simulink model "simulink_model_mbpo"  (R2022b)
settings: Solver=VariableStepAuto  StartTime=0.0  StopTime=5  FixedStep=1.0  RelTol=1e-3
values from neighbouring files (symbols this model uses):
  aa = (((m*l)^2)*g)/AA    (= 0.275046740282)    [createagent_mbpo.m]
  bb = (I +m*(l^2))*c/AA    (= 0.588785047389)    [createagent_mbpo.m]
  cc = (b*m*l)/AA    (= 4.42542074273e-05)    [createagent_mbpo.m]
  dd = (m*g*l*(M+m))/AA    (= 6.05102828621)    [createagent_mbpo.m]
  ee = (m*l*c)/AA    (= 0.353271042564)    [createagent_mbpo.m]
  ff = ((M+m)*b)/AA    (= 0.0009735925634)    [createagent_mbpo.m]
  mm = (I +m*(l^2))/AA    (= 0.9345794403)    [createagent_mbpo.m]
  nn = (m*l)/AA    (= 0.56074768661)    [createagent_mbpo.m]
  oo = (2*l)/AA    (= 11.2149537322)    [createagent_mbpo.m]
  thetastartdelta = 0    [createagent_mbpo.m]
  xstartdelta = 0    [createagent_mbpo.m]
libraries: rllib x1
settings Model: Creator=Wolfgang  LastModifiedBy=Wolfgang

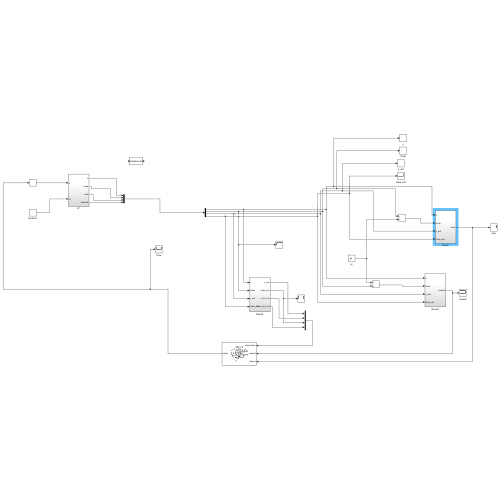
[thumbnail: Simulink's stored preview of the top-level diagram]
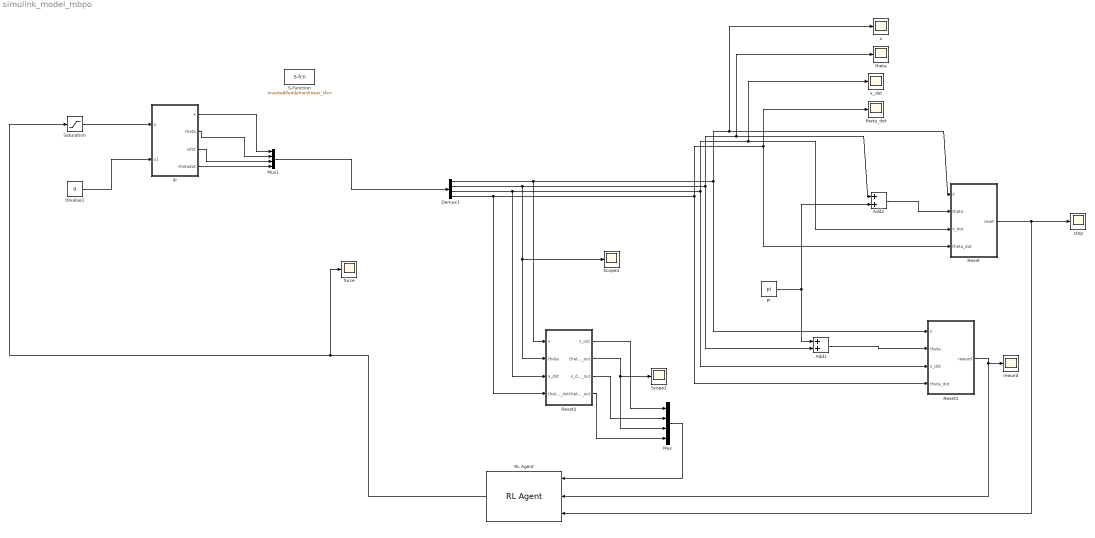
== system simulink_model_mbpo ==
  Add1 : Sum
  Add2 : Sum
  Demux1 : Demux
  IP : Subsystem
  Mux : Mux
  Mux1 : Mux
  RL Agent : rllib/RL Agent  Agent=agent  ExternalActionAsInput=off  ProvideLastAction=off  ProvideCumRwd=off  TreatAsDirectFeedthrough=on  UseStrictObservationDataTypes=off
  Reset : Subsystem
  Reset1 : Subsystem
  Reset2 : Subsystem
  S-Function : S-Function  FunctionName=invertedPendelnonlinear_sfcn  Parameters=xstart; thetastart; 0; 0  SFunctionDeploymentMode=off  EnableBusSupport=off
  Saturation : Saturate  UpperLimit=1000  LowerLimit=-1000
  Scope2 : Scope
  Scope4 : Scope
  force : Scope
  pi : Constant  Tag=tt  Value=pi
  reward : Scope
  stop : Scope
  t0value1 : Constant  Tag=tt  Value=0
  theta : Scope
  theta_dot : Scope
  x : Scope
  x_dot : Scope
  wires:
  Demux1/2 -> Scope4/1, Reset2/2(theta), Add1/2, Add2/1, theta/1
  Demux1/3 -> Reset2/3(x_dot), x_dot/1, Reset/3(x_dot), Reset1/3(x_dot)
  Demux1/4 -> Reset2/4(theta_dot), Reset/4(theta_dot), theta_dot/1, Reset1/4(theta_dot)
  Reset/1(reset) -> RL Agent/3, stop/1
  Reset1/1(reward) -> RL Agent/2, reward/1
  RL Agent/1 -> Saturation/1, force/1
  Mux/1 -> RL Agent/1
  Reset2/1(x_out) -> Mux/1
  Reset2/3(x_dot_out) -> Mux/2
  Reset2/2(theta_out) -> Scope2/1, Mux/3
  Reset2/4(theta_dot_out) -> Mux/4
  IP/1(x) -> Mux1/1
  Mux1/1 -> Demux1/1
  IP/3(xdot) -> Mux1/3
  IP/4(thetadot) -> Mux1/4
  t0value1/1 -> IP/2(u1)
  IP/2(theta) -> Mux1/2
  Demux1/1 -> Reset1/1(x), x/1, Reset/1(x), Reset2/1(x)
  Add1/1 -> Reset1/2(theta)
  Add2/1 -> Reset/2(theta)
  pi/1 -> Add2/2, Add1/1
  Saturation/1 -> IP/1(u)

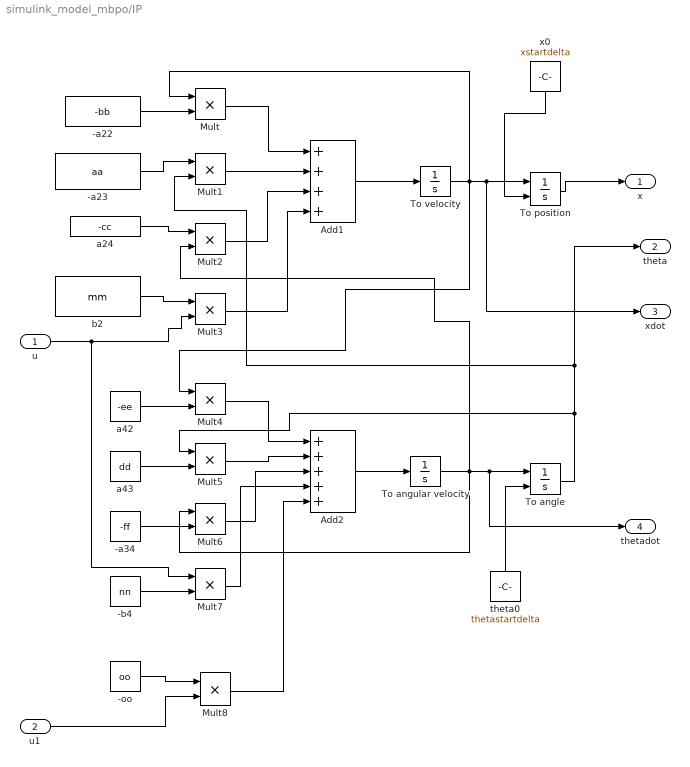
== system simulink_model_mbpo/IP ==
  u : Inport
  u1 : Inport  Port=2
  -a22 : Constant  Value=-bb
  -a23 : Constant  Value=aa
  -a34 : Constant  Value=-ff
  -b4 : Constant  Value=nn
  -oo : Constant  Value=oo
  Add1 : Sum  Inputs=++++
  Add2 : Sum  Inputs=+++++
  Mult{,1..8} (9 alike) : Product  Inputs=**
  To angle : Integrator  InitialConditionSource=external  InitialCondition=1.5
  To angular velocity : Integrator
  To position : Integrator  InitialConditionSource=external  InitialCondition=1
  To velocity : Integrator
  a24 : Constant  Value=-cc
  a42 : Constant  Value=-ee
  a43 : Constant  Value=dd
  b2 : Constant  Value=mm
  theta0 : Constant  Value=thetastartdelta
  x0 : Constant  Value=xstartdelta
  x : Outport  VectorParamsAs1DForOutWhenUnconnected=off
  theta : Outport  Port=2  VectorParamsAs1DForOutWhenUnconnected=off
  xdot : Outport  Port=3  VectorParamsAs1DForOutWhenUnconnected=off
  thetadot : Outport  Port=4  VectorParamsAs1DForOutWhenUnconnected=off
  wires:
  u1/1 -> Mult8/2
  -oo/1 -> Mult8/1
  Mult8/1 -> Add2/5
  x0/1 -> To position/2
  theta0/1 -> To angle/2
  To position/1 -> x/1
  a24/1 -> Mult2/1
  Mult5/1 -> Add2/2
  Mult/1 -> Add1/1
  a42/1 -> Mult4/2
  u/1 -> Mult3/2, Mult7/1
  Mult2/1 -> Add1/3
  Mult4/1 -> Add2/1
  a43/1 -> Mult5/2
  Mult7/1 -> Add2/4
  To angle/1 -> Mult5/1, Mult1/2, theta/1
  To velocity/1 -> To position/1, xdot/1, Mult/1, Mult4/1
  -a23/1 -> Mult1/1
  To angular velocity/1 -> To angle/1, thetadot/1, Mult2/2, Mult6/1
  b2/1 -> Mult3/1
  Add1/1 -> To velocity/1
  Mult1/1 -> Add1/2
  Mult3/1 -> Add1/4
  Mult6/1 -> Add2/3
  -b4/1 -> Mult7/2
  -a34/1 -> Mult6/2
  Add2/1 -> To angular velocity/1
  -a22/1 -> Mult/2

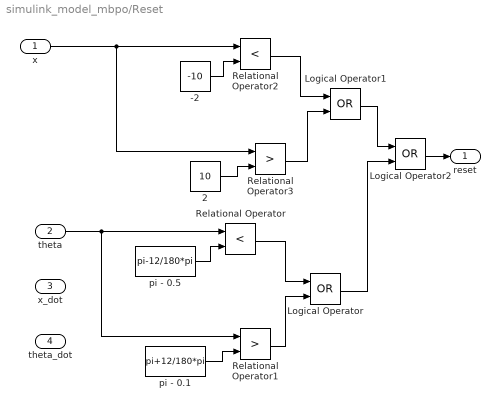
== system simulink_model_mbpo/Reset ==
  x : Inport
  theta : Inport  Port=2
  x_dot : Inport  Port=3
  theta_dot : Inport  Port=4
  -2 : Constant  Value=-10
  2 : Constant  Value=10
  Logical Operator : Logic  Operator=OR  AllPortsSameDT=off  OutDataTypeStr=boolean
  Logical Operator1 : Logic  Operator=OR  AllPortsSameDT=off  OutDataTypeStr=boolean
  Logical Operator2 : Logic  Operator=OR  AllPortsSameDT=off  OutDataTypeStr=boolean
  Relational Operator : RelationalOperator  Operator=<  OutDataTypeStr=boolean  RndMeth=Simplest  InputSameDT=off
  Relational Operator1 : RelationalOperator  Operator=>  OutDataTypeStr=boolean  RndMeth=Simplest  InputSameDT=off
  Relational Operator2 : RelationalOperator  Operator=<  OutDataTypeStr=boolean  RndMeth=Simplest  InputSameDT=off
  Relational Operator3 : RelationalOperator  Operator=>  OutDataTypeStr=boolean  RndMeth=Simplest  InputSameDT=off
  pi - 0.1 : Constant  Value=pi+12/180*pi
  pi - 0.5 : Constant  Value=pi-12/180*pi
  reset : Outport  VectorParamsAs1DForOutWhenUnconnected=off
  wires:
  theta/1 -> Relational Operator1/1, Relational Operator/1
  pi - 0.5/1 -> Relational Operator/2
  Relational Operator/1 -> Logical Operator/1
  pi - 0.1/1 -> Relational Operator1/2
  Logical Operator2/1 -> reset/1
  Relational Operator1/1 -> Logical Operator/2
  Relational Operator3/1 -> Logical Operator1/2
  Relational Operator2/1 -> Logical Operator1/1
  -2/1 -> Relational Operator2/2
  2/1 -> Relational Operator3/2
  x/1 -> Relational Operator3/1, Relational Operator2/1
  Logical Operator1/1 -> Logical Operator2/1
  Logical Operator/1 -> Logical Operator2/2

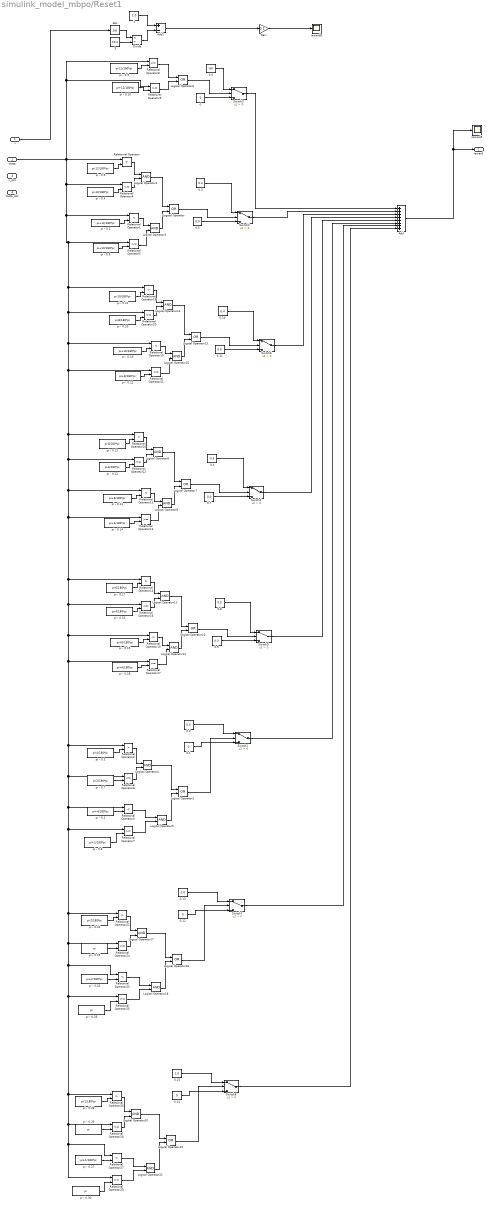
== system simulink_model_mbpo/Reset1 ==
  x : Inport
  theta : Inport  Port=2
  x_dot : Inport  Port=3
  theta_dot : Inport  Port=4
  -1 : Constant  Value=0
  0.1 : Constant  Value=0
  0.10 : Constant  Value=0.4
  0.{5,7,9,11} (4 alike) : Constant  Value=0.0
  0.12 : Constant  Value=0
  0.13 : Constant  Value=0.6
  0.14 : Constant  Value=0
  0.15 : Constant  Value=1.0
  0.2 : Constant  Value=0.5
  0.3 : Constant  Value=0.3
  0.4 : Constant  Value=0.5
  0.6 : Constant  Value=-50
  0.8 : Constant  Value=0.5
  1 : Constant  Value=1.0
  3 : Constant  Value=10.0
  Abs : Abs  SaturateOnIntegerOverflow=off
  Add : Sum  Inputs=++++++++
  Add1 : Sum  Inputs=+-
  Divide : Product  Inputs=*/
  Gain : Gain  Gain=0.1
  Logical Operator{,1,6..7,10,13,16,19} (8 alike) : Logic  Operator=OR  AllPortsSameDT=off  OutDataTypeStr=boolean
  Logical Operator{2..5,8..9,11..12,14..15,17..18,20..21} (14 alike) : Logic  AllPortsSameDT=off  OutDataTypeStr=boolean
  Relational Operator{,2,10,14,18,22,26} (7 alike) : RelationalOperator  Operator=>  OutDataTypeStr=boolean  RndMeth=Simplest  InputSameDT=off
  Relational Operator{1,3,11,15,19,23,27} (7 alike) : RelationalOperator  Operator=<  OutDataTypeStr=boolean  RndMeth=Simplest  InputSameDT=off
  Relational Operator{4,6,8,12,16,20,24,28} (8 alike) : RelationalOperator  Operator=<=  OutDataTypeStr=boolean  RndMeth=Simplest  InputSameDT=off
  Relational Operator{5,7,9,13,17,21,25,29} (8 alike) : RelationalOperator  OutDataTypeStr=boolean  RndMeth=Simplest  InputSameDT=off
  Switch{1..8} (8 alike) : Switch  Criteria=u2 > Threshold  SaturateOnIntegerOverflow=off  InputSameDT=off
  pi - 0.1 : Constant  Value=pi+12/180*pi
  pi - 0.10 : Constant  Value=pi+12/180*pi
  pi - 0.11 : Constant  Value=pi+8/180*pi
  pi - 0.12 : Constant  Value=pi-6/180*pi
  pi - 0.13 : Constant  Value=pi-8/180*pi
  pi - 0.14 : Constant  Value=pi+6/180*pi
  pi - 0.15 : Constant  Value=pi+6/180*pi
  pi - 0.16 : Constant  Value=pi-4/180*pi
  pi - 0.17 : Constant  Value=pi-6/180*pi
  pi - 0.18 : Constant  Value=pi+4/180*pi
  pi - 0.19 : Constant  Value=pi+10/180*pi
  pi - 0.2 : Constant  Value=pi+4/180*pi
  pi - 0.20 : Constant  Value=pi-8/180*pi
  pi - 0.21 : Constant  Value=pi-10/180*pi
  pi - 0.22 : Constant  Value=pi+8/180*pi
  pi - 0.23 : Constant  Value=pi+2/180*pi
  pi - 0.24 : Constant  Value=pi-2/180*pi
  pi - 0.{25..26,29..30} (4 alike) : Constant  Value=pi
  pi - 0.27 : Constant  Value=pi+1/180*pi
  pi - 0.28 : Constant  Value=pi-1/180*pi
  pi - 0.3 : Constant  Value=pi-4/180*pi
  pi - 0.4 : Constant  Value=pi-10/180*pi
  pi - 0.5 : Constant  Value=pi-12/180*pi
  pi - 0.6 : Constant  Value=pi+10/180*pi
  pi - 0.7 : Constant  Value=pi-2/180*pi
  pi - 0.8 : Constant  Value=pi+2/180*pi
  pi - 0.9 : Constant  Value=pi-12/180*pi
  reward5 : Scope
  reward8 : Scope
  reward : Outport  VectorParamsAs1DForOutWhenUnconnected=off
  wires:
  pi - 0.5/1 -> Relational Operator/2
  Relational Operator/1 -> Logical Operator2/1
  pi - 0.1/1 -> Relational Operator1/2
  pi - 0.2/1 -> Relational Operator3/2
  Relational Operator3/1 -> Logical Operator5/1
  pi - 0.3/1 -> Relational Operator2/2
  Logical Operator1/1 -> Switch1/2
  pi - 0.4/1 -> Relational Operator4/2
  Relational Operator4/1 -> Logical Operator2/2
  pi - 0.6/1 -> Relational Operator5/2
  Relational Operator5/1 -> Logical Operator3/2
  Relational Operator1/1 -> Logical Operator3/1
  Logical Operator3/1 -> Logical Operator/2
  Logical Operator2/1 -> Logical Operator/1
  pi - 0.7/1 -> Relational Operator6/2
  Relational Operator6/1 -> Logical Operator4/2
  Relational Operator2/1 -> Logical Operator4/1
  pi - 0.8/1 -> Relational Operator7/2
  Relational Operator7/1 -> Logical Operator5/2
  Logical Operator4/1 -> Logical Operator1/1
  Logical Operator5/1 -> Logical Operator1/2
  0.1/1 -> Switch1/3
  0.2/1 -> Switch1/1
  Logical Operator/1 -> Switch2/2
  0.5/1 -> Switch2/3
  0.3/1 -> Switch2/1
  pi - 0.9/1 -> Relational Operator8/2
  pi - 0.10/1 -> Relational Operator9/2
  Relational Operator9/1 -> Logical Operator6/2
  Relational Operator8/1 -> Logical Operator6/1
  Logical Operator6/1 -> Switch3/2
  -1/1 -> Switch3/3
  0.6/1 -> Switch3/1
  Switch3/1 -> Add/1
  Switch2/1 -> Add/2
  0.4/1 -> Switch4/1
  pi - 0.14/1 -> Relational Operator13/2
  Logical Operator8/1 -> Logical Operator7/1
  Logical Operator9/1 -> Logical Operator7/2
  Relational Operator11/1 -> Logical Operator9/1
  Relational Operator10/1 -> Logical Operator8/1
  Relational Operator13/1 -> Logical Operator9/2
  pi - 0.13/1 -> Relational Operator10/2
  pi - 0.11/1 -> Relational Operator11/2
  pi - 0.12/1 -> Relational Operator12/2
  Logical Operator7/1 -> Switch4/2
  0.7/1 -> Switch4/3
  Relational Operator12/1 -> Logical Operator8/2
  Relational Operator16/1 -> Logical Operator11/2
  Logical Operator10/1 -> Switch5/2
  pi - 0.15/1 -> Relational Operator15/2
  Relational Operator15/1 -> Logical Operator12/1
  Logical Operator12/1 -> Logical Operator10/2
  Relational Operator14/1 -> Logical Operator11/1
  Logical Operator11/1 -> Logical Operator10/1
  0.8/1 -> Switch5/1
  pi - 0.16/1 -> Relational Operator16/2
  pi - 0.17/1 -> Relational Operator14/2
  0.9/1 -> Switch5/3
  pi - 0.18/1 -> Relational Operator17/2
  Relational Operator17/1 -> Logical Operator12/2
  Relational Operator20/1 -> Logical Operator14/2
  Logical Operator13/1 -> Switch6/2
  pi - 0.20/1 -> Relational Operator20/2
  pi - 0.21/1 -> Relational Operator18/2
  pi - 0.19/1 -> Relational Operator19/2
  Relational Operator19/1 -> Logical Operator15/1
  Logical Operator15/1 -> Logical Operator13/2
  Relational Operator18/1 -> Logical Operator14/1
  Logical Operator14/1 -> Logical Operator13/1
  0.10/1 -> Switch6/1
  0.11/1 -> Switch6/3
  pi - 0.22/1 -> Relational Operator21/2
  Relational Operator21/1 -> Logical Operator15/2
  Switch6/1 -> Add/3
  Switch4/1 -> Add/4
  Switch5/1 -> Add/5
  Switch1/1 -> Add/6
  x/1 -> Abs/1
  1/1 -> Add1/1
  Abs/1 -> Divide/1
  3/1 -> Divide/2
  Divide/1 -> Add1/2
  Add1/1 -> Gain/1
  Gain/1 -> reward8/1
  Add/1 -> reward5/1, reward/1
  Logical Operator17/1 -> Logical Operator16/1
  Relational Operator24/1 -> Logical Operator17/2
  pi - 0.25/1 -> Relational Operator24/2
  pi - 0.26/1 -> Relational Operator25/2
  Logical Operator18/1 -> Logical Operator16/2
  0.12/1 -> Switch7/3
  Relational Operator22/1 -> Logical Operator17/1
  pi - 0.24/1 -> Relational Operator22/2
  pi - 0.23/1 -> Relational Operator23/2
  Logical Operator16/1 -> Switch7/2
  0.13/1 -> Switch7/1
  Relational Operator25/1 -> Logical Operator18/2
  Relational Operator23/1 -> Logical Operator18/1
  Switch7/1 -> Add/7
  Relational Operator26/1 -> Logical Operator20/1
  0.15/1 -> Switch8/1
  Relational Operator27/1 -> Logical Operator21/1
  Logical Operator19/1 -> Switch8/2
  Logical Operator21/1 -> Logical Operator19/2
  Relational Operator29/1 -> Logical Operator21/2
  pi - 0.28/1 -> Relational Operator26/2
  Logical Operator20/1 -> Logical Operator19/1
  0.14/1 -> Switch8/3
  pi - 0.30/1 -> Relational Operator29/2
  Relational Operator28/1 -> Logical Operator20/2
  pi - 0.29/1 -> Relational Operator28/2
  theta/1 -> Relational Operator/1, Relational Operator4/1, Relational Operator1/1, Relational Operator5/1, Relational Operator10/1, Relational Operator12/1, Relational Operator11/1, Relational Operator13/1, Relational Operator14/1, Relational Operator16/1, Relational Operator17/1, Relational Operator2/1, Relational Operator6/1, Relational Operator22/1, Relational Operator26/1, Relational Operator29/1, Relational Operator27/1, Relational Operator28/1, Relational Operator25/1, Relational Operator23/1, Relational Operator24/1, Relational Operator7/1, Relational Operator3/1, Relational Operator15/1, Relational Operator21/1, Relational Operator19/1, Relational Operator20/1, Relational Operator18/1, Relational Operator9/1, Relational Operator8/1
  pi - 0.27/1 -> Relational Operator27/2
  Switch8/1 -> Add/8

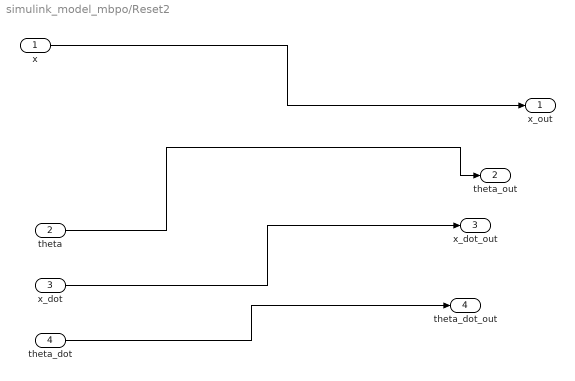
== system simulink_model_mbpo/Reset2 ==
  x : Inport
  theta : Inport  Port=2
  x_dot : Inport  Port=3
  theta_dot : Inport  Port=4
  x_out : Outport  VectorParamsAs1DForOutWhenUnconnected=off
  theta_out : Outport  Port=2  VectorParamsAs1DForOutWhenUnconnected=off
  x_dot_out : Outport  Port=3  VectorParamsAs1DForOutWhenUnconnected=off
  theta_dot_out : Outport  Port=4  VectorParamsAs1DForOutWhenUnconnected=off
  wires:
  theta/1 -> theta_out/1
  x/1 -> x_out/1
  x_dot/1 -> x_dot_out/1
  theta_dot/1 -> theta_dot_out/1
